simulink model "stdp"  (R2018a)
settings: Solver=VariableStepAuto  StartTime=0.0  StopTime=0.2  MaxStep=1e-6  RelTol=1e-3
libraries: fl_lib x5, nesl_utility x5, simulink x1
settings Model: Creator=bici  LastModifiedBy=bici
settings DataIOCC: SaveState=on  InspectSignalLogs=on
settings OptimizationCC: UseFloatMulNetSlope=on

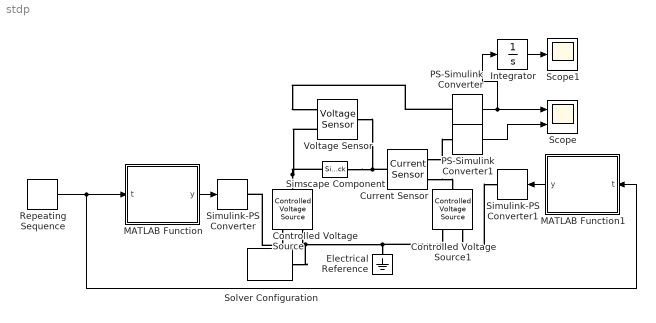
== system stdp ==
  Controlled Voltage Source : fl_lib/Electrical/Electrical Sources/Controlled Voltage Source
  Controlled Voltage Source1 : fl_lib/Electrical/Electrical Sources/Controlled Voltage Source
  Current Sensor : fl_lib/Electrical/Electrical Sensors/Current Sensor
  Electrical Reference : fl_lib/Electrical/Electrical Elements/Electrical Reference
  Integrator : Integrator
  MATLAB Function : MATLAB Function  TreatAsAtomicUnit=on  mask{A_p=1, A_n=0.25, tau_p=0.04, tau_n=0.003, t_p=0.005, t_n=0.075, zero=0.1001}
  MATLAB Function1 : MATLAB Function  TreatAsAtomicUnit=on  mask{A_p=1, A_n=0.25, tau_p=0.04, tau_n=0.003, t_p=0.005, t_n=0.075, zero=0.1}
  PS-Simulink Converter : nesl_utility/PS-Simulink Converter  PhysicalDomain=network_engine_domain  SubClassName=ps_output  LeftPortType=input  RightPortType=output  PseudoPeriodic=off  Frequencies=[]  Unit=1  AffineConversion=off
  PS-Simulink Converter1 : nesl_utility/PS-Simulink Converter  PhysicalDomain=network_engine_domain  SubClassName=ps_output  LeftPortType=input  RightPortType=output  PseudoPeriodic=off  Frequencies=[]  Unit=1  AffineConversion=off
  Repeating Sequence : simulink/Sources/Repeating Sequence  rep_seq_t=[0 0.2]  rep_seq_y=[0 0.2]
  Scope : Scope  NumInputPorts=2
  Scope1 : Scope
  Simscape Component : SimscapeComponentBlock  SourceFile=memristor_vteam_v2_exponential  ComponentPath=memristor_vteam_v2_exponential  ComponentVariants=memristor_vteam_v2_exponential  ComponentVariantNames=memristor_vteam_v2_exponential  ClassName=memristor_vteam_v2_exponential  SchemaVersion=1  k_off=5e-16 m/s  v_off=0.0015 V  a_off=3  k_on=-5e-16 m/s  v_on=-0.0015 V  a_on=3  R_off=100 Ohm  w_off=3e-9 m  R_on=10000 Ohm  w_on=0 m  i_specify=off  i_priority=None  i=0 A  i_nominal_specify=off  i_nominal_unit=A  i_nominal_value=1  v_specify=off  v_priority=None  v=0 V  v_nominal_specify=off  v_nominal_unit=V  v_nominal_value=1
      settings: CopyFcn=simscape.engine.sli.internal.componentblockcallback(gcbh,'COPY')  PreCopyFcn=simscape.engine.sli.internal.componentblockcallback(gcbh,'PRECOPY')  PreDeleteFcn=simscape.engine.sli.internal.componentblockcallback(gcbh,'PREDELETE')
      mask Type: memristor_vteam_v2_exponential
      mask Display:
      | disp('Simscape\n\n\n')
      | disp('\n\n\nmemristor_vteam_v2_exponential');
      | color('red');
      | port_label('RConn', 1,'-');
      | port_label('LConn', 1,'+');
  Simulink-PS Converter : nesl_utility/Simulink-PS Converter  PhysicalDomain=network_engine_domain  SubClassName=ps_input  LeftPortType=input  RightPortType=output  PseudoPeriodic=off  Frequencies=[]  NoiseDistribution=none  NoiseParameters=[]  Unit=1  AffineConversion=off  FilteringAndDerivatives=provide  SimscapeFilterOrder=1  InputFilterTimeConstant=0.001  UdotUserProvided=0
  Simulink-PS Converter1 : nesl_utility/Simulink-PS Converter  PhysicalDomain=network_engine_domain  SubClassName=ps_input  LeftPortType=input  RightPortType=output  PseudoPeriodic=off  Frequencies=[]  NoiseDistribution=none  NoiseParameters=[]  Unit=1  AffineConversion=off  FilteringAndDerivatives=provide  SimscapeFilterOrder=1  InputFilterTimeConstant=0.001  UdotUserProvided=0
  Solver Configuration : nesl_utility/Solver Configuration  PhysicalDomain=network_engine_domain  SubClassName=solver  LeftPortType=input  RightPortType=generic  Tones=[]  Harmonics=[]  SimulateNoise=off  Profile=off  UseLocalSampling=off  EnableSwitchedLinearOptims=on  FrequencyDomain=off  UseCCode=off  RelTol=0.001  AbsTol=1e-06  MinStep=1e-09  ToWorkspace=off  RevertToSquareIcSolve=off  NumHomotopyIterations=100  PhasorMode=off  PhasorModeNumHarmonics=1  DoDC=off  ResidualTolerance=1e-09  UseLocalSolver=off  LocalSolverChoice=NE_BACKWARD_EULER_ADVANCER  LocalSolverSampleTime=0.001  DoFixedCost=off  MaxNonlinIter=3  MaxModeIter=2  LinearAlgebra=Sparse  EquationFormulation=NE_TIME_EF  DelaysMemoryBudget=1024  AutomaticFiltering=on  FilteringTimeConstant=0.001
  Voltage Sensor : fl_lib/Electrical/Electrical Sensors/Voltage Sensor
  wires:
  MATLAB Function/1(y) -> Simulink-PS Converter/1
  Repeating Sequence/1 -> MATLAB Function1/1(t), MATLAB Function/1(t)
  PS-Simulink Converter/1 -> Integrator/1, Scope/1
  Integrator/1 -> Scope1/1
  MATLAB Function1/1(y) -> Simulink-PS Converter1/1
  PS-Simulink Converter1/1 -> Scope/2
  connections:
  Controlled Voltage Source/LConn1 -- Voltage Sensor/RConn2 -- Simscape Component/LConn1
  Voltage Sensor/LConn1 -- Current Sensor/LConn1 -- Simscape Component/RConn1
  Controlled Voltage Source/RConn2 -- Controlled Voltage Source1/RConn2 -- Electrical Reference/LConn1 -- Solver Configuration/RConn1
  PS-Simulink Converter/LConn1 -- Voltage Sensor/RConn1
  Controlled Voltage Source/RConn1 -- Simulink-PS Converter/RConn1
  Current Sensor/RConn2 -- Controlled Voltage Source1/LConn1
  Controlled Voltage Source1/RConn1 -- Simulink-PS Converter1/RConn1
  Current Sensor/RConn1 -- PS-Simulink Converter1/LConn1

== matlab function stdp/MATLAB Function1 ==
  data: t input; y output; A_p parameter; A_n parameter; tau_p parameter; tau_n parameter; t_p parameter; t_n parameter; zero parameter
function y = fcn(t, A_p, A_n, tau_p, tau_n, t_p, t_n, zero)

if ( (t>zero-t_p) && (t<zero) ) 
    y =  A_p*( exp((t-zero)/tau_p) - exp(-t_p/tau_p) ) / ( 1-exp(-t_p/tau_p) );
elseif ((t>zero) && (t<zero+t_n))
    y = -A_n*( exp(-(t-zero)/tau_n) - exp(-t_n/tau_n) ) / ( 1-exp(-t_n/tau_n) );
else
    y = 0;
end

== matlab function stdp/MATLAB Function ==
  data: t input; y output; A_p parameter; A_n parameter; tau_p parameter; tau_n parameter; t_p parameter; t_n parameter; zero parameter
function y = fcn(t, A_p, A_n, tau_p, tau_n, t_p, t_n, zero)

if ( (t>zero-t_p) && (t<zero) ) 
    y =  A_p*( exp((t-zero)/tau_p) - exp(-t_p/tau_p) ) / ( 1-exp(-t_p/tau_p) );
elseif ((t>zero) && (t<zero+t_n))
    y = -A_n*( exp(-(t-zero)/tau_n) - exp(-t_n/tau_n) ) / ( 1-exp(-t_n/tau_n) );
else
    y = 0;
end
